simulink model "Pre_SysGen_Post_sh_fifo_nohwcs"  (Simulink 10.0)
settings: Solver=ode45  StartTime=0.0  StopTime=500000  RelTol=1e-3
InitFcn:
  | init
undefined symbols (not defined in the file): blk, cols, fps, rows
libraries: xbsIndex_r4 x178, simulink x14, dspbuff3 x6, dspmtrx3 x3, vipsnks x2, dspsrcs4 x2, dspsigops x1, dspwin32 x1
(part 1 of 2)
settings Model: Creator=ahwang  LastModifiedBy=bhisma
settings DataIOCC: LimitDataPoints=on  SignalLoggingSaveFormat=ModelDataLogs
settings OptimizationCC: ExpressionDepthLimit=2147483647  InitFltsAndDblsToZero=on
settings DebuggingCC: SaveWithParameterizedLinksMsg=none  SolverPrmCheckMsg=warning  FcnCallInpInsideContextMsg=warning  StateNameClashWarn=warning
settings SFSimCC: SimUseLocalCustomCode=on  CustomCodeUndefinedFunction=FilterOut
settings RTWCC: RTWUseLocalCustomCode=on
settings GRTTargetCC: TargetFcnLib=ansi_tfl_tmw.mat

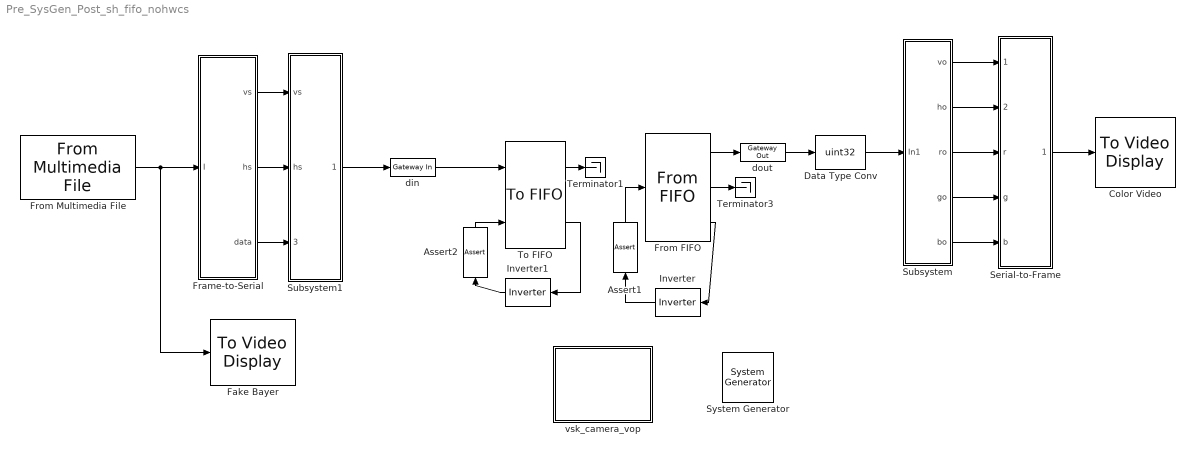
== system Pre_SysGen_Post_sh_fifo_nohwcs ==
  " System Generator" : xbsIndex_r4/ System Generator  Tag=genX  SystemSampleTime=-1  xilinxfamily=spartan3adsp  part=xc3sd1800a  speed=-4  package=fg676  synthesis_tool=XST  directory=./netlist  testbench=off  simulink_period=1  sysclk_period=20  incr_netlist=off  trim_vbits=Everywhere in SubSystem  dbl_ovrd=According to Block Masks  core_generation=According to Block Masks  run_coregen=off  deprecated_control=off  eval_field=0  block_type=sysgen
      settings: block_version=9.2.01
  Assert1 : xbsIndex_r4/Assert  assert_type=off  type_source=Explicitly  arith_type=Unsigned  n_bits=8  bin_pt=2  assert_rate=on  rate_source=Explicitly  period=1  output_port=on  block_type=assert
      settings: infoedit=Asserts a user-defined sample rate and/or type on a signal.  block_version=VER_STRING_GOES_HERE
  Assert2 : xbsIndex_r4/Assert  assert_type=off  type_source=Explicitly  arith_type=Unsigned  n_bits=8  bin_pt=2  assert_rate=on  rate_source=Explicitly  period=1  output_port=on  block_type=assert
      settings: infoedit=Asserts a user-defined sample rate and/or type on a signal.  block_version=VER_STRING_GOES_HERE
  Color Video : vipsnks/To Video Display  inputType=Obsolete  imagePorts=One multidimensional signal  OutputDevice=On-screen video monitor  fullScreen=off  videoWindowX=559  videoWindowY=678  saveWindowSize=off  videoWindowWidth=44  videoWindowHeight=41  dataOrg=Column-major
      settings: SourceProductName=Computer Vision Toolbox  SourceProductBaseCode=VP
  Data Type Conv : DataTypeConversion  OutDataTypeStr=uint32
  Fake Bayer : vipsnks/To Video Display  inputType=Obsolete  imagePorts=One multidimensional signal  OutputDevice=On-screen video monitor  fullScreen=off  videoWindowX=177  videoWindowY=679  saveWindowSize=off  videoWindowWidth=44  videoWindowHeight=41  dataOrg=Column-major
      settings: SourceProductName=Computer Vision Toolbox  SourceProductBaseCode=VP
  Frame-to-Serial : Subsystem
  From FIFO : xbsIndex_r4/From FIFO  shared_memory_name='data_out'  ownership=Owned elsewhere  depth=4K  percent_nbits=8  has_arst=off  arith_type=Unsigned  n_bits=32  bin_pt=0  dbl_ovrd=off  mem_type=Block RAM  block_type=fromfifo
      settings: AttributesFormatString=<< %<shared_memory_name> >>  infoedit=First-in-first-out (FIFO) block that reads FIFO data from shared memory storage.  block_version=VER_STRING_GOES_HERE
  From Multimedia File : dspwin32/From Multimedia File  inputFilename=C:\hill\WWM\seminars\mathworks_vsk\seminar_designs\viptrain_gbrg.avi  loop=on  numPlays=inf  outputStreams=Video only  videoDataType=uint8  audioDataType=int16  inheritSampleTime=off  userDefinedSampleTime=1/fps  noAudioOutput=off  isIntensityVideo=on  colorVideoFormat=One multidimensional signal  outputEOF=off  dataOrg=Column-major
      settings: SourceProductName=DSP System Toolbox  SourceProductBaseCode=DS
  Inverter : xbsIndex_r4/Inverter  en=off  latency=0  dbl_ovrd=off  block_type=inv
      settings: block_version=VER_STRING_GOES_HERE
  Inverter1 : xbsIndex_r4/Inverter  en=off  latency=0  dbl_ovrd=off  block_type=inv
      settings: block_version=VER_STRING_GOES_HERE
  Serial-to-Frame : Subsystem
  Subsystem : Subsystem
  Subsystem1 : Subsystem
  Terminator1 : Terminator
  Terminator3 : Terminator
  To FIFO : xbsIndex_r4/To FIFO  shared_memory_name='data_in'  ownership=Owned elsewhere  depth=16  percent_nbits=1  has_arst=off  explicit_data_type=on  arith_type=Unsigned  n_bits=16  bin_pt=0  dbl_ovrd=off  mem_type=Block RAM  block_type=tofifo
      settings: AttributesFormatString=<< %<shared_memory_name> >>  infoedit=First-in-first-out (FIFO) block that writes FIFO data to shared memory storage.  block_version=VER_STRING_GOES_HERE
  din : xbsIndex_r4/Gateway In  arith_type=Unsigned  n_bits=16  bin_pt=0  quantization="Round  (unbiased: +/- Inf)"  overflow=Saturate  period=1  dbl_ovrd=off  timing_constraint=None  locs_specified=off  LOCs={}  block_type=gatewayin
      settings: infoedit="Gateway in block.  Converts inputs of type Simulink integer, double and fixed point to  Xilinx fixed point type.<P><P>Hardware notes:  In hardware these blocks become top level input ports."  xl_area=[0, 0, 0, 0, 0, 0, 0]  block_version=VER_STRING_GOES_HERE
  dout : xbsIndex_r4/Gateway Out  hdl_port=on  timing_constraint=None  locs_specified=off  LOCs={}  block_type=gatewayout
      settings: infoedit="Gateway out block.  Converts Xilinx fixed point inputs into ouputs of type Simulink integer, double, or fixed point.<P><P>Hardware notes:  In hardware these blocks become top level output ports or are discarded, depending on how they are configured."  xl_area=[0, 0, 0, 0, 0, 0, 0]  block_version=VER_STRING_GOES_HERE
  vsk_camera_vop : Subsystem
  wires:
  From Multimedia File/1 -> Frame-to-Serial/1(I), Fake Bayer/1
  Serial-to-Frame/1(v_out) -> Color Video/1
  Frame-to-Serial/3(data) -> Subsystem1/3(data)
  Frame-to-Serial/2(hs) -> Subsystem1/2(hs)
  Frame-to-Serial/1(vs) -> Subsystem1/1(vs)
  Subsystem/5(bo) -> Serial-to-Frame/5(b)
  Subsystem/4(go) -> Serial-to-Frame/4(g)
  Subsystem/2(ho) -> Serial-to-Frame/2(hsync)
  Subsystem/1(vo) -> Serial-to-Frame/1(vsync)
  Subsystem/3(ro) -> Serial-to-Frame/3(r)
  From FIFO/1 -> dout/1
  din/1 -> To FIFO/1
  To FIFO/1 -> Terminator1/1
  To FIFO/2 -> Inverter1/1
  From FIFO/2 -> Terminator3/1
  From FIFO/3 -> Inverter/1
  Inverter/1 -> Assert1/1
  Assert2/1 -> To FIFO/2
  Assert1/1 -> From FIFO/1
  Inverter1/1 -> Assert2/1
  Subsystem1/1(Out1) -> din/1
  dout/1 -> Data Type Conv/1
  Data Type Conv/1 -> Subsystem/1(In1)

== system Pre_SysGen_Post_sh_fifo_nohwcs/Frame-to-Serial ==
  I : Inport
  Math Function : Math  Operator=transpose  SaturateOnIntegerOverflow=on
  Subsystem1 : Subsystem
  vs : Outport
  hs : Outport  Port=2
  data : Outport  Port=3
  wires:
  I/1 -> Math Function/1
  Math Function/1 -> Subsystem1/1(I)
  Subsystem1/1(vs) -> vs/1
  Subsystem1/2(hs) -> hs/1
  Subsystem1/3(data) -> data/1

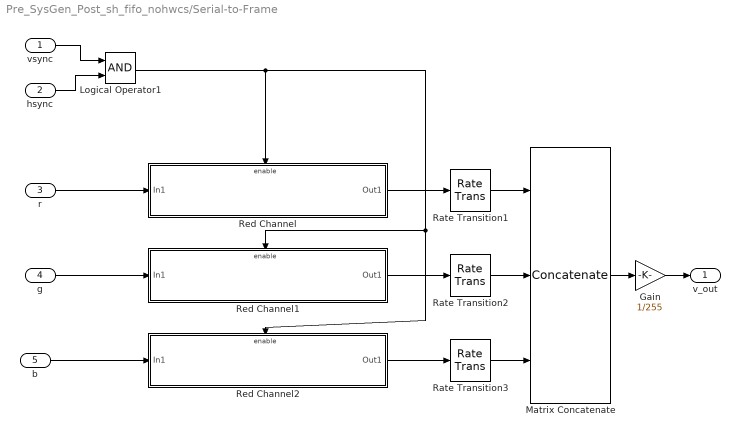
== system Pre_SysGen_Post_sh_fifo_nohwcs/Serial-to-Frame ==
  vsync : Inport
  hsync : Inport  Port=2
  r : Inport  Port=3
  g : Inport  Port=4
  b : Inport  Port=5
  Gain : Gain  Gain=1/255
  Logical Operator1 : Logic  AllPortsSameDT=off  OutDataTypeStr=boolean
  Matrix Concatenate : Concatenate  NumInputs=3  Mode=Multidimensional array  ConcatenateDimension=3
  Rate Transition1 : RateTransition  Deterministic=off  OutPortSampleTime=1/fps
  Rate Transition2 : RateTransition  Deterministic=off  OutPortSampleTime=1/fps
  Rate Transition3 : RateTransition  Deterministic=off  OutPortSampleTime=1/fps
  Red Channel : Subsystem
  Red Channel1 : Subsystem
  Red Channel2 : Subsystem
  v_out : Outport
  wires:
  Matrix Concatenate/1 -> Gain/1
  r/1 -> Red Channel/1(In1)
  g/1 -> Red Channel1/1(In1)
  b/1 -> Red Channel2/1(In1)
  Red Channel/1(Out1) -> Rate Transition1/1
  Red Channel1/1(Out1) -> Rate Transition2/1
  Red Channel2/1(Out1) -> Rate Transition3/1
  vsync/1 -> Logical Operator1/1
  hsync/1 -> Logical Operator1/2
  Logical Operator1/1 -> Red Channel/Enable, Red Channel1/Enable, Red Channel2/Enable
  Rate Transition1/1 -> Matrix Concatenate/1
  Rate Transition2/1 -> Matrix Concatenate/2
  Rate Transition3/1 -> Matrix Concatenate/3
  Gain/1 -> v_out/1

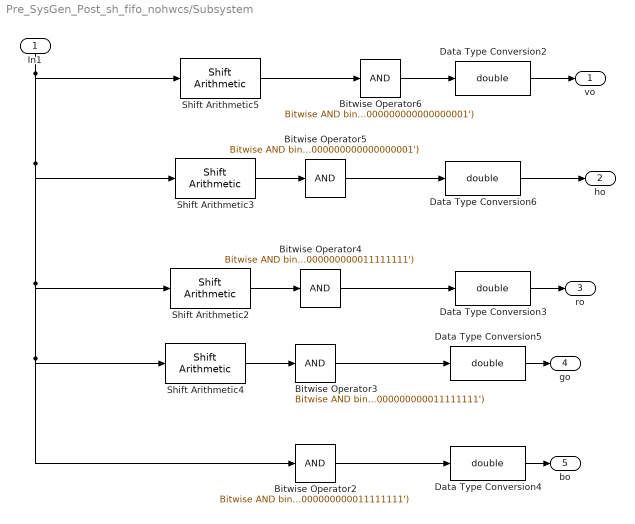
== system Pre_SysGen_Post_sh_fifo_nohwcs/Subsystem ==
  In1 : Inport
  Bitwise Operator2 : simulink/Logic and Bit Operations/Bitwise Operator  logicop=AND  UseBitMask=on  BitMask=bin2dec('000000000000000000011111111')  BitMaskRealWorld=Stored Integer
  Bitwise Operator3 : simulink/Logic and Bit Operations/Bitwise Operator  logicop=AND  UseBitMask=on  BitMask=bin2dec('000000000000000000011111111')  BitMaskRealWorld=Stored Integer
  Bitwise Operator4 : simulink/Logic and Bit Operations/Bitwise Operator  logicop=AND  UseBitMask=on  BitMask=bin2dec('000000000000000000011111111')  BitMaskRealWorld=Stored Integer
  Bitwise Operator5 : simulink/Logic and Bit Operations/Bitwise Operator  logicop=AND  UseBitMask=on  BitMask=bin2dec('000000000000000000000000001')  BitMaskRealWorld=Stored Integer
  Bitwise Operator6 : simulink/Logic and Bit Operations/Bitwise Operator  logicop=AND  UseBitMask=on  BitMask=bin2dec('000000000000000000000000001')  BitMaskRealWorld=Stored Integer
  Data Type Conversion{2..6} (5 alike) : DataTypeConversion  OutDataTypeStr=double
  Shift Arithmetic2 : simulink/Logic and Bit Operations/Shift Arithmetic  SystemSampleTime=-1  nBitShiftRight=16  nBinPtShiftRight=0
      settings: SourceProductName=Simulink  SourceProductBaseCode=SL
  Shift Arithmetic3 : simulink/Logic and Bit Operations/Shift Arithmetic  SystemSampleTime=-1  nBitShiftRight=24  nBinPtShiftRight=0
      settings: SourceProductName=Simulink  SourceProductBaseCode=SL
  Shift Arithmetic4 : simulink/Logic and Bit Operations/Shift Arithmetic  SystemSampleTime=-1  nBitShiftRight=8  nBinPtShiftRight=0
      settings: SourceProductName=Simulink  SourceProductBaseCode=SL
  Shift Arithmetic5 : simulink/Logic and Bit Operations/Shift Arithmetic  SystemSampleTime=-1  nBitShiftRight=25  nBinPtShiftRight=0
      settings: SourceProductName=Simulink  SourceProductBaseCode=SL
  vo : Outport
  ho : Outport  Port=2
  ro : Outport  Port=3
  go : Outport  Port=4
  bo : Outport  Port=5
  wires:
  Bitwise Operator5/1 -> Data Type Conversion6/1
  Bitwise Operator4/1 -> Data Type Conversion3/1
  Bitwise Operator3/1 -> Data Type Conversion5/1
  Shift Arithmetic5/1 -> Bitwise Operator6/1
  Shift Arithmetic3/1 -> Bitwise Operator5/1
  Shift Arithmetic2/1 -> Bitwise Operator4/1
  Shift Arithmetic4/1 -> Bitwise Operator3/1
  Bitwise Operator2/1 -> Data Type Conversion4/1
  In1/1 -> Shift Arithmetic5/1, Shift Arithmetic3/1, Shift Arithmetic2/1, Shift Arithmetic4/1, Bitwise Operator2/1
  Bitwise Operator6/1 -> Data Type Conversion2/1
  Data Type Conversion6/1 -> ho/1
  Data Type Conversion3/1 -> ro/1
  Data Type Conversion5/1 -> go/1
  Data Type Conversion4/1 -> bo/1
  Data Type Conversion2/1 -> vo/1

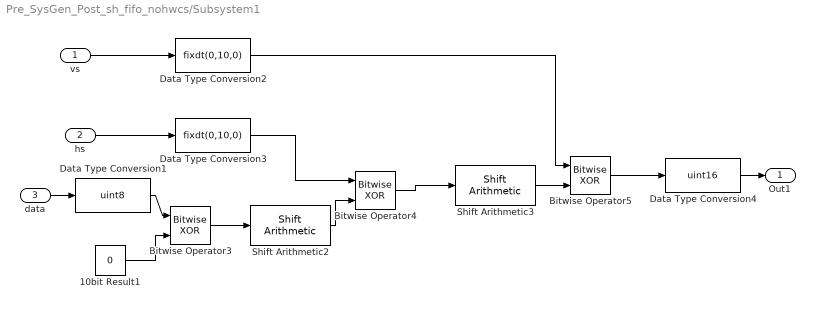
== system Pre_SysGen_Post_sh_fifo_nohwcs/Subsystem1 ==
  vs : Inport
  hs : Inport  Port=2
  data : Inport  Port=3
  10bit Result1 : Constant  Value=0  OutDataTypeStr=fixdt(0,10,0)
  Bitwise Operator3 : simulink/Logic and Bit Operations/Bitwise Operator  logicop=XOR  UseBitMask=off  NumInputPorts=2  BitMask=bin2dec('11011001')  BitMaskRealWorld=Stored Integer
  Bitwise Operator4 : simulink/Logic and Bit Operations/Bitwise Operator  logicop=XOR  UseBitMask=off  NumInputPorts=2  BitMask=bin2dec('11011001')  BitMaskRealWorld=Stored Integer
  Bitwise Operator5 : simulink/Logic and Bit Operations/Bitwise Operator  logicop=XOR  UseBitMask=off  NumInputPorts=2  BitMask=bin2dec('11011001')  BitMaskRealWorld=Stored Integer
  Data Type Conversion1 : DataTypeConversion  OutDataTypeStr=uint8
  Data Type Conversion2 : DataTypeConversion  OutDataTypeStr=fixdt(0,10,0)
  Data Type Conversion3 : DataTypeConversion  OutDataTypeStr=fixdt(0,10,0)
  Data Type Conversion4 : DataTypeConversion  OutDataTypeStr=uint16
  Shift Arithmetic2 : simulink/Logic and Bit Operations/Shift Arithmetic  SystemSampleTime=-1  nBitShiftRight=-1  nBinPtShiftRight=0
      settings: SourceProductName=Simulink  SourceProductBaseCode=SL
  Shift Arithmetic3 : simulink/Logic and Bit Operations/Shift Arithmetic  SystemSampleTime=-1  nBitShiftRight=-1  nBinPtShiftRight=0
      settings: SourceProductName=Simulink  SourceProductBaseCode=SL
  Out1 : Outport
  wires:
  10bit Result1/1 -> Bitwise Operator3/2
  Bitwise Operator3/1 -> Shift Arithmetic2/1
  Bitwise Operator4/1 -> Shift Arithmetic3/1
  Data Type Conversion1/1 -> Bitwise Operator3/1
  Shift Arithmetic2/1 -> Bitwise Operator4/2
  Data Type Conversion3/1 -> Bitwise Operator4/1
  Data Type Conversion2/1 -> Bitwise Operator5/1
  Shift Arithmetic3/1 -> Bitwise Operator5/2
  vs/1 -> Data Type Conversion2/1
  hs/1 -> Data Type Conversion3/1
  Bitwise Operator5/1 -> Data Type Conversion4/1
  data/1 -> Data Type Conversion1/1
  Data Type Conversion4/1 -> Out1/1

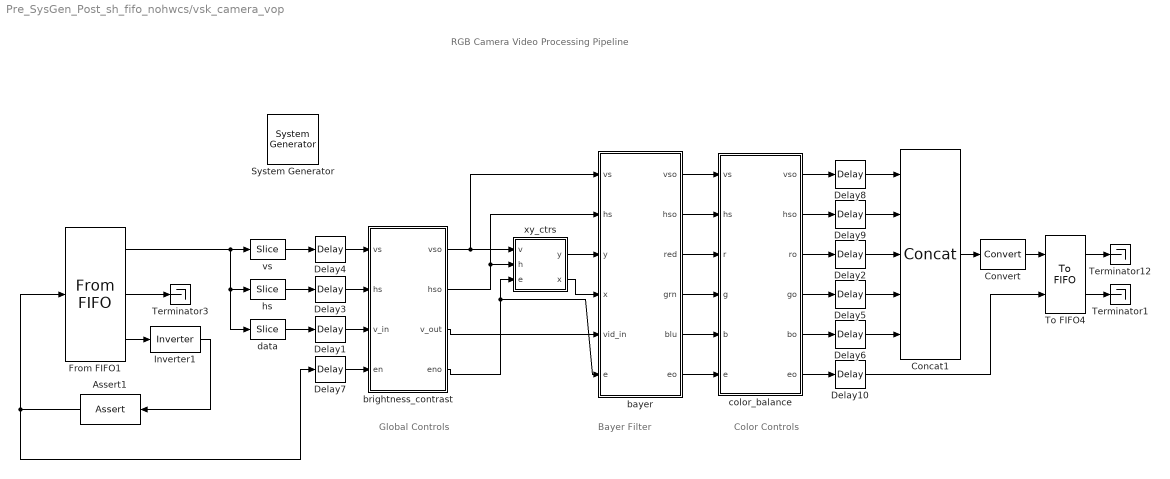
== system Pre_SysGen_Post_sh_fifo_nohwcs/vsk_camera_vop ==
  note: Color
      | Controls
  note: Global
      | Controls
  note: Bayer Filter
  note: RGB Camera Video Processing Pipeline
  " System Generator" : xbsIndex_r4/ System Generator  Tag=genX  SystemSampleTime=-1  xilinxfamily=spartan3adsp  part=xc3sd1800a  speed=-4  package=fg676  synthesis_tool=XST  directory=./netlist  testbench=off  simulink_period=1  sysclk_period=20  incr_netlist=off  trim_vbits=Everywhere in SubSystem  dbl_ovrd=According to Block Masks  core_generation=According to Block Masks  run_coregen=off  deprecated_control=off  eval_field=0  block_type=sysgen
      settings: block_version=9.2.01
  Assert1 : xbsIndex_r4/Assert  assert_type=off  type_source=Explicitly  arith_type=Unsigned  n_bits=8  bin_pt=2  assert_rate=on  rate_source=Explicitly  period=1  output_port=on  block_type=assert
      settings: infoedit=Asserts a user-defined sample rate and/or type on a signal.  block_version=VER_STRING_GOES_HERE
  Concat1 : xbsIndex_r4/Concat  num_inputs=5  dbl_ovrd=off  block_type=concat
      settings: block_version=9.2.01
  Convert : xbsIndex_r4/Convert  arith_type=Unsigned  n_bits=32  bin_pt=0  quantization=Truncate  overflow=Wrap  latency=0  dbl_ovrd=off  pipeline=off  block_type=convert
      settings: block_version=9.2.01
  Delay{1,3..4,7} (4 alike) : xbsIndex_r4/Delay  en=off  latency=20  dbl_ovrd=off  reg_retiming=on  block_type=delay
      settings: infoedit="Delay line having  configurable length.<P><P>Hardware notes: A delay line is a chain, each link of which is an SRL16 followed by a flip-flop. If register retiming is enabled, the delay line is a chain of flip-flops."  xl_area=[0, 0, 0, 0, 0, 0, 0]  block_version=VER_STRING_GOES_HERE
  Delay{2,5..6,8..10} (6 alike) : xbsIndex_r4/Delay  en=off  latency=1  dbl_ovrd=off  reg_retiming=on  block_type=delay
      settings: infoedit="Delay line having  configurable length.<P><P>Hardware notes: A delay line is a chain, each link of which is an SRL16 followed by a flip-flop. If register retiming is enabled, the delay line is a chain of flip-flops."  xl_area=[0, 0, 0, 0, 0, 0, 0]  block_version=VER_STRING_GOES_HERE
  From FIFO1 : xbsIndex_r4/From FIFO  shared_memory_name='data_in'  ownership=Locally owned  depth=64K  percent_nbits=1  has_arst=off  arith_type=Unsigned  n_bits=16  bin_pt=0  dbl_ovrd=off  mem_type=Block RAM  block_type=fromfifo
      settings: AttributesFormatString=<< %<shared_memory_name> >>  infoedit=First-in-first-out (FIFO) block that reads FIFO data from shared memory storage.  block_version=VER_STRING_GOES_HERE
  Inverter1 : xbsIndex_r4/Inverter  en=off  latency=0  dbl_ovrd=off  block_type=inv
      settings: block_version=VER_STRING_GOES_HERE
  Terminator1 : Terminator
  Terminator12 : Terminator
  Terminator3 : Terminator
  To FIFO4 : xbsIndex_r4/To FIFO  shared_memory_name='data_out'  ownership=Locally owned  depth=64K  percent_nbits=1  has_arst=off  explicit_data_type=on  arith_type=Unsigned  n_bits=32  bin_pt=0  dbl_ovrd=off  mem_type=Block RAM  block_type=tofifo
      settings: AttributesFormatString=<< %<shared_memory_name> >>  infoedit=First-in-first-out (FIFO) block that writes FIFO data to shared memory storage.  block_version=VER_STRING_GOES_HERE
  bayer : Subsystem
  brightness_contrast : Subsystem
  color_balance : Subsystem
  data : xbsIndex_r4/Slice  nbits=8  boolean_output=off  mode=Lower Bit Location + Width  bit1=0  base1=MSB of Input  bit0=2  base0=LSB of Input  dbl_ovrd=off  block_type=slice
      settings: infoedit="Extracts a given range of bits from each input sample and presents it at the output.  The output type is ordinarily unsigned with binary point at zero, but can be Boolean when the slice is one bit wide.<P><P>Hardware notes: In hardware this block costs nothing."  block_version=9.2.01
  hs : xbsIndex_r4/Slice  nbits=1  boolean_output=off  mode=Lower Bit Location + Width  bit1=0  base1=MSB of Input  bit0=1  base0=LSB of Input  dbl_ovrd=off  block_type=slice
      settings: infoedit="Extracts a given range of bits from each input sample and presents it at the output.  The output type is ordinarily unsigned with binary point at zero, but can be Boolean when the slice is one bit wide.<P><P>Hardware notes: In hardware this block costs nothing."  block_version=9.2.01
  vs : xbsIndex_r4/Slice  nbits=1  boolean_output=off  mode=Lower Bit Location + Width  bit1=0  base1=MSB of Input  bit0=0  base0=LSB of Input  dbl_ovrd=off  block_type=slice
      settings: infoedit="Extracts a given range of bits from each input sample and presents it at the output.  The output type is ordinarily unsigned with binary point at zero, but can be Boolean when the slice is one bit wide.<P><P>Hardware notes: In hardware this block costs nothing."  block_version=9.2.01
  xy_ctrs : Subsystem
  wires:
  Delay1/1 -> brightness_contrast/3(v_in)
  Delay3/1 -> brightness_contrast/2(hs)
  Delay4/1 -> brightness_contrast/1(vs)
  bayer/2(hso) -> color_balance/2(hs)
  bayer/1(vso) -> color_balance/1(vs)
  color_balance/2(hso) -> Delay9/1
  color_balance/1(vso) -> Delay8/1
  brightness_contrast/2(hso) -> bayer/2(hs), xy_ctrs/2(h)
  brightness_contrast/4(eno) -> xy_ctrs/3(e), bayer/6(e)
  brightness_contrast/1(vso) -> xy_ctrs/1(v), bayer/1(vs)
  Delay7/1 -> brightness_contrast/4(en)
  xy_ctrs/2(x) -> bayer/4(x)
  xy_ctrs/1(y) -> bayer/3(y)
  color_balance/5(bo) -> Delay6/1
  color_balance/4(go) -> Delay5/1
  color_balance/3(ro) -> Delay2/1
  bayer/6(eo) -> color_balance/6(e)
  bayer/5(blu) -> color_balance/5(b)
  bayer/4(grn) -> color_balance/4(g)
  bayer/3(red) -> color_balance/3(r)
  brightness_contrast/3(v_out) -> bayer/5(vid_in)
  From FIFO1/2 -> Terminator3/1
  From FIFO1/3 -> Inverter1/1
  From FIFO1/1 -> hs/1, data/1, vs/1
  To FIFO4/1 -> Terminator12/1
  vs/1 -> Delay4/1
  hs/1 -> Delay3/1
  data/1 -> Delay1/1
  To FIFO4/2 -> Terminator1/1
  Delay6/1 -> Concat1/5
  Delay5/1 -> Concat1/4
  Delay2/1 -> Concat1/3
  Delay9/1 -> Concat1/2
  Delay8/1 -> Concat1/1
  Concat1/1 -> Convert/1
  Inverter1/1 -> Assert1/1
  Assert1/1 -> From FIFO1/1, Delay7/1
  Convert/1 -> To FIFO4/1
  color_balance/6(eo) -> Delay10/1
  Delay10/1 -> To FIFO4/2

== system Pre_SysGen_Post_sh_fifo_nohwcs/Frame-to-Serial/Subsystem1 ==
  I : Inport
  Add : Sum
  Delay : dspsigops/Delay  dly_unit=Samples  delay=1  ic_detail=off  dif_ic_for_ch=off  dif_ic_for_dly=off  ic=0  reset_popup=Falling edge
      settings: SourceProductName=DSP System Toolbox  SourceProductBaseCode=DS
  Enabled Subsystem : Subsystem  TreatAsAtomicUnit=on
  Logical Operator : Logic  AllPortsSameDT=off  OutDataTypeStr=boolean
  Reshape : Reshape
  hsync : dspsrcs4/Signal From Workspace  SystemSampleTime=-1  X=[zeros(1,blk) ones(1,cols) zeros(1,blk)]  Ts=(1/fps)/ (rows*(cols+2*blk))  nsamps=1  OutputAfterFinalValue=Cyclic repetition  ignoreOrWarnInputAndFrameLengths=off
  vsync : dspsrcs4/Signal From Workspace  SystemSampleTime=-1  X=[ zeros(1,blk) ones(1,rows*(cols+2*blk)-2*blk) zeros(1,blk) ]  Ts=(1/fps)/(rows*(cols+2*blk))  nsamps=1  OutputAfterFinalValue=Cyclic repetition  ignoreOrWarnInputAndFrameLengths=off
  vs : Outport
  hs : Outport  Port=2
  data : Outport  Port=3
  wires:
  I/1 -> Reshape/1
  vsync/1 -> Delay/2, vs/1, Logical Operator/1  "Frame Valid"
  hsync/1 -> Add/2, hs/1, Logical Operator/2  "Line Valid"
  Delay/1 -> Add/1
  Add/1 -> Delay/1, Enabled Subsystem/2(Idx)
  Enabled Subsystem/1(Out1) -> data/1
  Reshape/1 -> Enabled Subsystem/1(I)
  Logical Operator/1 -> Enabled Subsystem/Enable

== system Pre_SysGen_Post_sh_fifo_nohwcs/Serial-to-Frame/Red Channel ==
  In1 : Inport
  Enable : EnablePort
  Buffer : dspbuff3/Buffer  N=cols  V=0  ic=0
      settings: SourceProductName=DSP System Toolbox  SourceProductBaseCode=DS
  Buffer1 : dspbuff3/Buffer  N=rows  V=0  ic=0
      settings: SourceProductName=DSP System Toolbox  SourceProductBaseCode=DS
  Frame Conversion1 : FrameConversion  OutFrame=Sample-based
  Matrix Concatenate : Concatenate  Mode=Multidimensional array
  Selector : Selector  NumberOfDimensions=2  InputPortWidth=3  IndexOptions=Index vector (dialog),Select all  Indices=22:rows,1  OutputSizes=1,1
  Selector1 : Selector  NumberOfDimensions=2  InputPortWidth=3  IndexOptions=Index vector (dialog),Select all  Indices=1:21,1  OutputSizes=1,1
  Transpose : dspmtrx3/Transpose  SystemSampleTime=-1  Hermitian=off  overflowFlag=off
      settings: SourceProductName=DSP System Toolbox  SourceProductBaseCode=DS
  Out1 : Outport
  wires:
  Buffer/1 -> Transpose/1
  In1/1 -> Buffer/1
  Transpose/1 -> Buffer1/1
  Frame Conversion1/1 -> Out1/1
  Matrix Concatenate/1 -> Frame Conversion1/1
  Selector/1 -> Matrix Concatenate/1
  Selector1/1 -> Matrix Concatenate/2
  Buffer1/1 -> Selector1/1, Selector/1

== system Pre_SysGen_Post_sh_fifo_nohwcs/Serial-to-Frame/Red Channel1 ==
  In1 : Inport
  Enable : EnablePort
  Buffer : dspbuff3/Buffer  N=cols  V=0  ic=0
      settings: SourceProductName=DSP System Toolbox  SourceProductBaseCode=DS
  Buffer1 : dspbuff3/Buffer  N=rows  V=0  ic=0
      settings: SourceProductName=DSP System Toolbox  SourceProductBaseCode=DS
  Frame Conversion1 : FrameConversion  OutFrame=Sample-based
  Matrix Concatenate : Concatenate  Mode=Multidimensional array
  Selector : Selector  NumberOfDimensions=2  InputPortWidth=3  IndexOptions=Index vector (dialog),Select all  Indices=22:rows,1  OutputSizes=1,1
  Selector1 : Selector  NumberOfDimensions=2  InputPortWidth=3  IndexOptions=Index vector (dialog),Select all  Indices=1:21,1  OutputSizes=1,1
  Transpose : dspmtrx3/Transpose  SystemSampleTime=-1  Hermitian=off  overflowFlag=off
      settings: SourceProductName=DSP System Toolbox  SourceProductBaseCode=DS
  Out1 : Outport
  wires:
  Buffer1/1 -> Selector/1, Selector1/1
  Selector1/1 -> Matrix Concatenate/2
  Selector/1 -> Matrix Concatenate/1
  Matrix Concatenate/1 -> Frame Conversion1/1
  Frame Conversion1/1 -> Out1/1
  Transpose/1 -> Buffer1/1
  In1/1 -> Buffer/1
  Buffer/1 -> Transpose/1

== system Pre_SysGen_Post_sh_fifo_nohwcs/Serial-to-Frame/Red Channel2 ==
  In1 : Inport
  Enable : EnablePort
  Buffer : dspbuff3/Buffer  N=cols  V=0  ic=0
      settings: SourceProductName=DSP System Toolbox  SourceProductBaseCode=DS
  Buffer1 : dspbuff3/Buffer  N=rows  V=0  ic=0
      settings: SourceProductName=DSP System Toolbox  SourceProductBaseCode=DS
  Frame Conversion1 : FrameConversion  OutFrame=Sample-based
  Matrix Concatenate : Concatenate  Mode=Multidimensional array
  Selector : Selector  NumberOfDimensions=2  InputPortWidth=3  IndexOptions=Index vector (dialog),Select all  Indices=22:rows,1  OutputSizes=1,1
  Selector1 : Selector  NumberOfDimensions=2  InputPortWidth=3  IndexOptions=Index vector (dialog),Select all  Indices=1:21,1  OutputSizes=1,1
  Transpose : dspmtrx3/Transpose  SystemSampleTime=-1  Hermitian=off  overflowFlag=off
      settings: SourceProductName=DSP System Toolbox  SourceProductBaseCode=DS
  Out1 : Outport
  wires:
  Buffer/1 -> Transpose/1
  In1/1 -> Buffer/1
  Transpose/1 -> Buffer1/1
  Frame Conversion1/1 -> Out1/1
  Matrix Concatenate/1 -> Frame Conversion1/1
  Selector/1 -> Matrix Concatenate/1
  Selector1/1 -> Matrix Concatenate/2
  Buffer1/1 -> Selector1/1, Selector/1

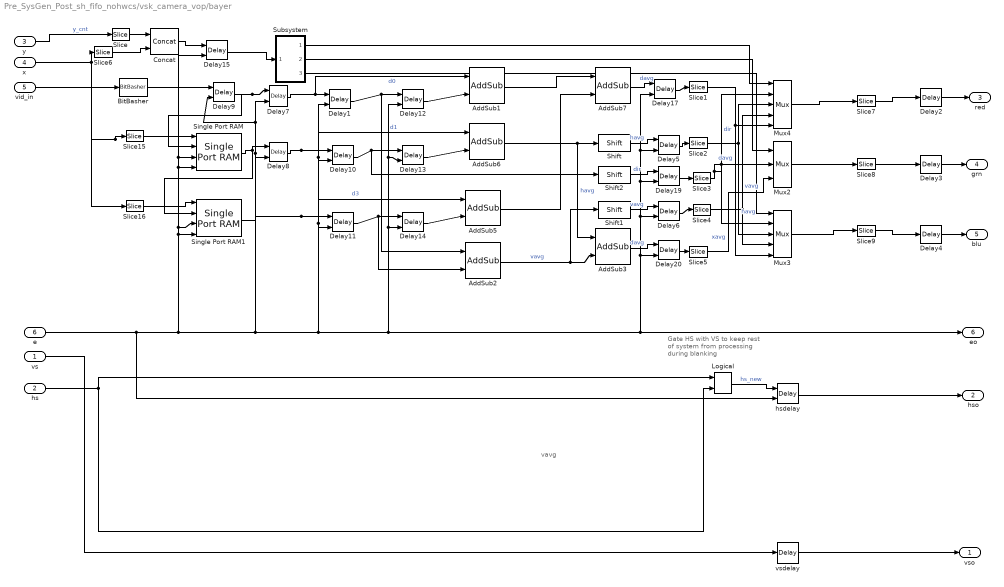
== system Pre_SysGen_Post_sh_fifo_nohwcs/vsk_camera_vop/bayer ==
  note: Gate HS with VS to keep
      | rest of system from
      | processing during blanking
  note: vavg
  vs : Inport
  hs : Inport  Port=2
  y : Inport  Port=3
  x : Inport  Port=4
  vid_in : Inport  Port=5
  e : Inport  Port=6
  AddSub{1..3,5..7} (6 alike) : xbsIndex_r4/AddSub  mode=Addition  use_carryin=off  use_carryout=off  en=off  latency=0  precision=Full  arith_type=Unsigned  n_bits=8  bin_pt=2  quantization=Truncate  overflow=Wrap  dbl_ovrd=off  use_behavioral_HDL=off  pipelined=off  use_rpm=on  block_type=addsub
      settings: xl_area=[0, 0, 0, 0, 0, 0, 0]  block_version=VER_STRING_GOES_HERE
  BitBasher : xbsIndex_r4/BitBasher  bitexpr=|  display_expr=off  sr_1=1  arith_type1=Unsigned  bin_pt1=0  sr_2=2  arith_type2=Unsigned  bin_pt2=0  sr_3=3  arith_type3=Unsigned  bin_pt3=0  sr_4=4  arith_type4=Unsigned  bin_pt4=0  dbl_ovrd=off  block_type=bitbasher
      | <html><head><meta name="qrichtext" content="1" /><style type="text/css">
      | p, li { white-space: pre-wrap; }
      | </style></head><body style=" font-family:'MS Shell Dlg 2'; font-size:8.25pt; font-weight:400; font-style:normal;">
      | <p style=" margin-top:12px; margin-bottom:12px; margin-left:0px; margin-right:0px; -qt-block-indent:0; text-indent:0px; font-family:'MS Shell Dlg'; font-size:8pt;">pad={in,2'b00}</p></body></html>
      settings: block_version=9.2.01
  Concat : xbsIndex_r4/Concat  num_inputs=2  dbl_ovrd=off  block_type=concat
      settings: block_version=VER_STRING_GOES_HERE
  Delay{1,5..6,8,10..15,17,19..20} (13 alike) : xbsIndex_r4/Delay  en=on  latency=1  dbl_ovrd=off  reg_retiming=on  block_type=delay
      settings: infoedit="Delay line having  configurable length.<P><P>Hardware notes: A delay line is a chain, each link of which is an SRL16 followed by a flip-flop. If register retiming is enabled, the delay line is a chain of flip-flops."  xl_area=[0, 0, 0, 0, 0, 0, 0]  block_version=VER_STRING_GOES_HERE
  Delay2 : xbsIndex_r4/Delay  en=off  latency=1  dbl_ovrd=off  reg_retiming=on  block_type=delay
      settings: infoedit="Delay line having  configurable length.<P><P>Hardware notes: A delay line is a chain, each link of which is an SRL16 followed by a flip-flop. If register retiming is enabled, the delay line is a chain of flip-flops."  xl_area=[0, 0, 0, 0, 0, 0, 0]  block_version=VER_STRING_GOES_HERE
  Delay3 : xbsIndex_r4/Delay  en=off  latency=1  dbl_ovrd=off  reg_retiming=on  block_type=delay
      settings: infoedit="Delay line having  configurable length.<P><P>Hardware notes: A delay line is a chain, each link of which is an SRL16 followed by a flip-flop. If register retiming is enabled, the delay line is a chain of flip-flops."  xl_area=[0, 0, 0, 0, 0, 0, 0]  block_version=VER_STRING_GOES_HERE
  Delay4 : xbsIndex_r4/Delay  en=off  latency=1  dbl_ovrd=off  reg_retiming=on  block_type=delay
      settings: infoedit="Delay line having  configurable length.<P><P>Hardware notes: A delay line is a chain, each link of which is an SRL16 followed by a flip-flop. If register retiming is enabled, the delay line is a chain of flip-flops."  xl_area=[0, 0, 0, 0, 0, 0, 0]  block_version=VER_STRING_GOES_HERE
  Delay7 : xbsIndex_r4/Delay  en=on  latency=2  dbl_ovrd=off  reg_retiming=on  block_type=delay
      settings: infoedit="Delay line having  configurable length.<P><P>Hardware notes: A delay line is a chain, each link of which is an SRL16 followed by a flip-flop. If register retiming is enabled, the delay line is a chain of flip-flops."  xl_area=[0, 0, 0, 0, 0, 0, 0]  block_version=VER_STRING_GOES_HERE
  Delay9 : xbsIndex_r4/Delay  en=on  latency=2  dbl_ovrd=off  reg_retiming=on  block_type=delay
      settings: infoedit="Delay line having  configurable length.<P><P>Hardware notes: A delay line is a chain, each link of which is an SRL16 followed by a flip-flop. If register retiming is enabled, the delay line is a chain of flip-flops."  xl_area=[0, 0, 0, 0, 0, 0, 0]  block_version=VER_STRING_GOES_HERE
  Logical : xbsIndex_r4/Logical  logical_function=AND  inputs=2  en=off  latency=0  precision=Full  arith_type=Unsigned  n_bits=16  bin_pt=0  align_bp=on  dbl_ovrd=off  block_type=logical
      settings: block_version=9.2.01
  Mux2 : xbsIndex_r4/Mux  inputs=2  en=off  latency=0  precision=Full  arith_type="Signed  (2's comp)"  n_bits=8  bin_pt=2  quantization=Truncate  overflow=Wrap  dbl_ovrd=off  block_type=mux
      settings: xl_area=[0, 0, 0, 0, 0, 0, 0]  block_version=VER_STRING_GOES_HERE
  Mux3 : xbsIndex_r4/Mux  inputs=4  en=off  latency=0  precision=Full  arith_type="Signed  (2's comp)"  n_bits=8  bin_pt=2  quantization=Truncate  overflow=Wrap  dbl_ovrd=off  block_type=mux
      settings: xl_area=[0, 0, 0, 0, 0, 0, 0]  block_version=VER_STRING_GOES_HERE
  Mux4 : xbsIndex_r4/Mux  inputs=4  en=off  latency=0  precision=Full  arith_type="Signed  (2's comp)"  n_bits=8  bin_pt=2  quantization=Truncate  overflow=Wrap  dbl_ovrd=off  block_type=mux
      settings: xl_area=[0, 0, 0, 0, 0, 0, 0]  block_version=VER_STRING_GOES_HERE
  Shift : xbsIndex_r4/Shift  shift_dir=Left  shift_bits=1  en=off  latency=0  precision=User Defined  arith_type=Unsigned  n_bits=12  bin_pt=0  quantization=Truncate  overflow=Wrap  dbl_ovrd=off  block_type=shift
      settings: xl_area=[0, 0, 0, 0, 0, 0, 0]  block_version=VER_STRING_GOES_HERE
  Shift1 : xbsIndex_r4/Shift  shift_dir=Left  shift_bits=1  en=off  latency=0  precision=User Defined  arith_type=Unsigned  n_bits=12  bin_pt=0  quantization=Truncate  overflow=Wrap  dbl_ovrd=off  block_type=shift
      settings: xl_area=[0, 0, 0, 0, 0, 0, 0]  block_version=VER_STRING_GOES_HERE
  Shift2 : xbsIndex_r4/Shift  shift_dir=Left  shift_bits=2  en=off  latency=0  precision=User Defined  arith_type=Unsigned  n_bits=12  bin_pt=0  quantization=Truncate  overflow=Wrap  dbl_ovrd=off  block_type=shift
      settings: xl_area=[0, 0, 0, 0, 0, 0, 0]  block_version=VER_STRING_GOES_HERE
  Single Port RAM : xbsIndex_r4/Single Port RAM  depth=1024  initVector=0  distributed_mem=Block RAM  write_mode=Read Before Write  rst=off  init_reg=0  en=on  latency=1  dbl_ovrd=off  optimize=Area  use_rpm=off  block_type=spram
      settings: xl_area=[0, 0, 0, 0, 0, 0, 0]  block_version=8.2
  Single Port RAM1 : xbsIndex_r4/Single Port RAM  depth=1024  initVector=0  distributed_mem=Block RAM  write_mode=Read Before Write  rst=off  init_reg=0  en=on  latency=1  dbl_ovrd=off  optimize=Area  use_rpm=off  block_type=spram
      settings: xl_area=[0, 0, 0, 0, 0, 0, 0]  block_version=8.2
  Slice : xbsIndex_r4/Slice  nbits=1  boolean_output=off  mode=Lower Bit Location + Width  bit1=0  base1=MSB of Input  bit0=0  base0=LSB of Input  dbl_ovrd=off  block_type=slice
      settings: infoedit="Extracts a given range of bits from each input sample and presents it at the output.  The output type is ordinarily unsigned with binary point at zero, but can be Boolean when the slice is one bit wide.<P><P>Hardware notes: In hardware this block costs nothing."  block_version=VER_STRING_GOES_HERE
  Slice{1..5} (5 alike) : xbsIndex_r4/Slice  nbits=10  boolean_output=off  mode=Lower Bit Location + Width  bit1=0  base1=MSB of Input  bit0=2  base0=LSB of Input  dbl_ovrd=off  block_type=slice
      settings: infoedit="Extracts a given range of bits from each input sample and presents it at the output.  The output type is ordinarily unsigned with binary point at zero, but can be Boolean when the slice is one bit wide.<P><P>Hardware notes: In hardware this block costs nothing."  block_version=VER_STRING_GOES_HERE
  Slice15 : xbsIndex_r4/Slice  nbits=10  boolean_output=off  mode=Lower Bit Location + Width  bit1=0  base1=MSB of Input  bit0=0  base0=LSB of Input  dbl_ovrd=off  block_type=slice
      settings: infoedit="Extracts a given range of bits from each input sample and presents it at the output.  The output type is ordinarily unsigned with binary point at zero, but can be Boolean when the slice is one bit wide.<P><P>Hardware notes: In hardware this block costs nothing."  block_version=VER_STRING_GOES_HERE
  Slice16 : xbsIndex_r4/Slice  nbits=10  boolean_output=off  mode=Lower Bit Location + Width  bit1=0  base1=MSB of Input  bit0=0  base0=LSB of Input  dbl_ovrd=off  block_type=slice
      settings: infoedit="Extracts a given range of bits from each input sample and presents it at the output.  The output type is ordinarily unsigned with binary point at zero, but can be Boolean when the slice is one bit wide.<P><P>Hardware notes: In hardware this block costs nothing."  block_version=VER_STRING_GOES_HERE
  Slice6 : xbsIndex_r4/Slice  nbits=1  boolean_output=off  mode=Lower Bit Location + Width  bit1=0  base1=MSB of Input  bit0=0  base0=LSB of Input  dbl_ovrd=off  block_type=slice
      settings: infoedit="Extracts a given range of bits from each input sample and presents it at the output.  The output type is ordinarily unsigned with binary point at zero, but can be Boolean when the slice is one bit wide.<P><P>Hardware notes: In hardware this block costs nothing."  block_version=VER_STRING_GOES_HERE
  Slice7 : xbsIndex_r4/Slice  nbits=8  boolean_output=off  mode=Lower Bit Location + Width  bit1=0  base1=MSB of Input  bit0=2  base0=LSB of Input  dbl_ovrd=off  block_type=slice
      settings: infoedit="Extracts a given range of bits from each input sample and presents it at the output.  The output type is ordinarily unsigned with binary point at zero, but can be Boolean when the slice is one bit wide.<P><P>Hardware notes: In hardware this block costs nothing."  block_version=VER_STRING_GOES_HERE
  Slice8 : xbsIndex_r4/Slice  nbits=8  boolean_output=off  mode=Lower Bit Location + Width  bit1=0  base1=MSB of Input  bit0=2  base0=LSB of Input  dbl_ovrd=off  block_type=slice
      settings: infoedit="Extracts a given range of bits from each input sample and presents it at the output.  The output type is ordinarily unsigned with binary point at zero, but can be Boolean when the slice is one bit wide.<P><P>Hardware notes: In hardware this block costs nothing."  block_version=VER_STRING_GOES_HERE
  Slice9 : xbsIndex_r4/Slice  nbits=8  boolean_output=off  mode=Lower Bit Location + Width  bit1=0  base1=MSB of Input  bit0=2  base0=LSB of Input  dbl_ovrd=off  block_type=slice
      settings: infoedit="Extracts a given range of bits from each input sample and presents it at the output.  The output type is ordinarily unsigned with binary point at zero, but can be Boolean when the slice is one bit wide.<P><P>Hardware notes: In hardware this block costs nothing."  block_version=VER_STRING_GOES_HERE
  Subsystem : Subsystem
  hsdelay : xbsIndex_r4/Delay  en=on  latency=7  dbl_ovrd=off  reg_retiming=on  block_type=delay
      settings: infoedit="Delay line having  configurable length.<P><P>Hardware notes: A delay line is a chain, each link of which is an SRL16 followed by a flip-flop. If register retiming is enabled, the delay line is a chain of flip-flops."  xl_area=[0, 0, 0, 0, 0, 0, 0]  block_version=VER_STRING_GOES_HERE
  vsdelay : xbsIndex_r4/Delay  en=off  latency=7  dbl_ovrd=off  reg_retiming=on  block_type=delay
      settings: infoedit="Delay line having  configurable length.<P><P>Hardware notes: A delay line is a chain, each link of which is an SRL16 followed by a flip-flop. If register retiming is enabled, the delay line is a chain of flip-flops."  xl_area=[0, 0, 0, 0, 0, 0, 0]  block_version=VER_STRING_GOES_HERE
  vso : Outport
  hso : Outport  Port=2
  red : Outport  Port=3
  grn : Outport  Port=4
  blu : Outport  Port=5
  eo : Outport  Port=6
  wires:
  Logical/1 -> hsdelay/1  "hs_new"
  vs/1 -> vsdelay/1
  e/1 -> hsdelay/2, Single Port RAM1/4, Delay15/2, Single Port RAM/3, Single Port RAM/4, Single Port RAM1/3, Delay10/2, Delay1/2, Delay11/2, Delay20/2, Delay6/2, Delay19/2, Delay5/2, Delay17/2, eo/1, Delay13/2, Delay12/2, Delay14/2, Delay7/2, Delay9/2, Delay8/2
  hs/1 -> Logical/1, Logical/2
  Slice9/1 -> Delay4/1
  Slice8/1 -> Delay3/1
  Slice7/1 -> Delay2/1
  vid_in/1 -> BitBasher/1
  BitBasher/1 -> Delay9/1
  Slice4/1 -> Mux3/4, Mux4/4  "vavg"
  Slice2/1 -> Mux3/3, Mux4/3  "havg"
  Slice1/1 -> Mux3/5, Mux4/5  "davg"
  Concat/1 -> Delay15/1
  Delay15/1 -> Subsystem/1(pos)
  Slice6/1 -> Concat/2
  Slice/1 -> Concat/1
  Slice5/1 -> Mux2/3  "xavg"
  Slice3/1 -> Mux3/2, Mux2/2, Mux4/2  "dir"
  Delay8/1 -> AddSub6/1, Delay10/1  "d1"
  Delay7/1 -> AddSub1/1, Delay1/1  "d0"
  x/1 -> Slice6/1, Slice15/1, Slice16/1
  Shift2/1 -> Delay19/1  "dir"
  Shift1/1 -> Delay6/1  "vavg"
  Shift/1 -> Delay5/1  "havg"
  Delay20/1 -> Slice5/1
  AddSub3/1 -> Delay20/1  "davg"
  Delay5/1 -> Slice2/1
  Delay19/1 -> Slice3/1
  Delay6/1 -> Slice4/1
  AddSub2/1 -> Shift1/1, AddSub3/2  "vavg"
  Subsystem/2(gsel) -> Mux2/1
  Slice16/1 -> Single Port RAM1/1
  Slice15/1 -> Single Port RAM/1
  Subsystem/1(rsel) -> Mux4/1
  Delay4/1 -> blu/1
  Delay3/1 -> grn/1
  Delay2/1 -> red/1
  Mux3/1 -> Slice9/1
  Mux2/1 -> Slice8/1
  Mux4/1 -> Slice7/1
  Subsystem/3(bsel) -> Mux3/1
  y/1 -> Slice/1  "y_cnt"
  AddSub6/1 -> Shift/1, AddSub3/1  "havg"
  Delay17/1 -> Slice1/1
  AddSub7/1 -> Delay17/1  "davg"
  AddSub5/1 -> AddSub7/2
  AddSub1/1 -> AddSub7/1
  Delay13/1 -> AddSub6/2
  Delay14/1 -> AddSub5/2
  Delay12/1 -> AddSub1/2
  Delay11/1 -> AddSub2/2, Delay14/1
  Delay10/1 -> Shift2/1, Delay13/1
  Delay1/1 -> AddSub2/1, Delay12/1
  Single Port RAM1/1 -> AddSub5/1, Delay11/1  "d3"
  Delay9/1 -> Delay7/1, Single Port RAM/2
  Single Port RAM/1 -> Single Port RAM1/2, Delay8/1
  hsdelay/1 -> hso/1
  vsdelay/1 -> vso/1

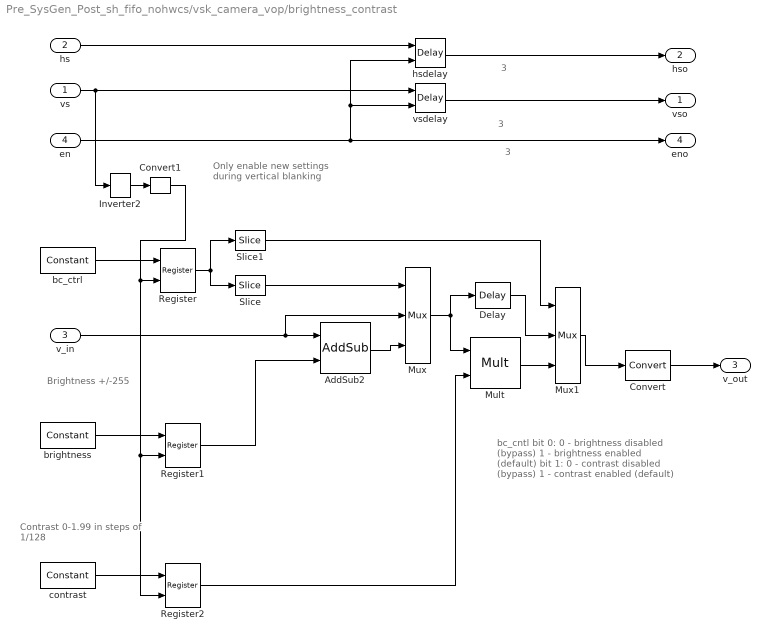
== system Pre_SysGen_Post_sh_fifo_nohwcs/vsk_camera_vop/brightness_contrast ==
  note: Only enable new settings
      | during vertical blanking
  note: bc_cntl
      | bit 0: 0 - brightness disabled (bypass)
      | 1 - brightness enabled (default)
      | bit 1: 0 - contrast disabled (bypass)
      | 1 - contrast enabled (default)
  note: Contrast
      | 0-1.99 in steps of 1/128
  note: Brightness
      | +/-255
  note: 3
  note: 3
  note: 3
  vs : Inport
  hs : Inport  Port=2
  v_in : Inport  Port=3
  en : Inport  Port=4
  AddSub2 : xbsIndex_r4/AddSub  mode=Addition  use_carryin=off  use_carryout=off  en=off  latency=0  precision=Full  arith_type=Unsigned  n_bits=8  bin_pt=2  quantization=Truncate  overflow=Wrap  dbl_ovrd=off  use_behavioral_HDL=off  pipelined=off  use_rpm=on  block_type=addsub
      settings: xl_area=[0, 0, 0, 0, 0, 0, 0]  block_version=VER_STRING_GOES_HERE
  Convert : xbsIndex_r4/Convert  arith_type=Unsigned  n_bits=8  bin_pt=0  quantization="Round  (unbiased: +/- Inf)"  overflow=Saturate  latency=0  dbl_ovrd=off  pipeline=off  block_type=convert
      settings: block_version=9.2.01
  Convert1 : xbsIndex_r4/Convert  arith_type=Boolean  n_bits=16  bin_pt=14  quantization=Truncate  overflow=Wrap  latency=0  dbl_ovrd=off  pipeline=off  block_type=convert
      settings: block_version=9.2.01
  Delay : xbsIndex_r4/Delay  en=off  latency=3  dbl_ovrd=off  reg_retiming=off  block_type=delay
      settings: block_version=9.2.01
  Inverter2 : xbsIndex_r4/Inverter  en=off  latency=0  dbl_ovrd=off  block_type=inv
      settings: block_version=9.2.01
  Mult : xbsIndex_r4/Mult  precision=Full  arith_type="Signed  (2's comp)"  n_bits=8  bin_pt=2  quantization=Truncate  overflow=Wrap  en=off  latency=3  dbl_ovrd=off  use_behavioral_HDL=off  use_embedded=on  opt=Speed  optimum_pipeline=off  pipeline=on  use_rpm=on  placement_style=Rectangular shape  block_type=mult
      settings: infoedit=Multiplies two values.<P><P>Hardware notes: To use the internal pipeline stage of the dedicated multiplier you must select 'Pipeline to Greatest Extent Possible'.  xl_area=[0, 0, 0, 0, 0, 0, 0]  block_version=VER_STRING_GOES_HERE
  Mux : xbsIndex_r4/Mux  inputs=2  en=off  latency=0  precision=Full  arith_type=Unsigned  n_bits=16  bin_pt=14  quantization=Truncate  overflow=Wrap  dbl_ovrd=off  block_type=mux
      settings: block_version=9.2.01
  Mux1 : xbsIndex_r4/Mux  inputs=2  en=off  latency=0  precision=Full  arith_type=Unsigned  n_bits=16  bin_pt=14  quantization=Truncate  overflow=Wrap  dbl_ovrd=off  block_type=mux
      settings: block_version=9.2.01
  Register : xbsIndex_r4/Register  init=0  rst=off  en=on  dbl_ovrd=off  block_type=register
      settings: block_version=9.2.01
  Register1 : xbsIndex_r4/Register  init=0  rst=off  en=on  dbl_ovrd=off  block_type=register
      settings: block_version=9.2.01
  Register2 : xbsIndex_r4/Register  init=0  rst=off  en=on  dbl_ovrd=off  block_type=register
      settings: block_version=9.2.01
  Slice : xbsIndex_r4/Slice  nbits=1  boolean_output=off  mode=Lower Bit Location + Width  bit1=0  base1=MSB of Input  bit0=0  base0=LSB of Input  dbl_ovrd=off  block_type=slice
      settings: infoedit="Extracts a given range of bits from each input sample and presents it at the output.  The output type is ordinarily unsigned with binary point at zero, but can be Boolean when the slice is one bit wide.<P><P>Hardware notes: In hardware this block costs nothing."  block_version=9.2.01
  Slice1 : xbsIndex_r4/Slice  nbits=1  boolean_output=off  mode=Lower Bit Location + Width  bit1=0  base1=MSB of Input  bit0=1  base0=LSB of Input  dbl_ovrd=off  block_type=slice
      settings: infoedit="Extracts a given range of bits from each input sample and presents it at the output.  The output type is ordinarily unsigned with binary point at zero, but can be Boolean when the slice is one bit wide.<P><P>Hardware notes: In hardware this block costs nothing."  block_version=9.2.01
  bc_ctrl : xbsIndex_r4/Constant  arith_type=Unsigned  const=0  n_bits=9  bin_pt=0  explicit_period=off  period=1  equ=P=C  opselect=C  inp2=PCIN>>17  opr=+  inp1=P  carry=CIN  dbl_ovrd=off  block_type=constant
      settings: block_version=9.2.01
  brightness : xbsIndex_r4/Constant  arith_type=Signed (2's comp)  const=0  n_bits=9  bin_pt=0  explicit_period=off  period=1  equ=P=C  opselect=C  inp2=PCIN>>17  opr=+  inp1=P  carry=CIN  dbl_ovrd=off  block_type=constant
      settings: block_version=9.2.01
  contrast : xbsIndex_r4/Constant  arith_type=Unsigned  const=8  n_bits=7  bin_pt=0  explicit_period=off  period=1  equ=P=C  opselect=C  inp2=PCIN>>17  opr=+  inp1=P  carry=CIN  dbl_ovrd=off  block_type=constant
      settings: block_version=9.2.01
  hsdelay : xbsIndex_r4/Delay  en=on  latency=3  dbl_ovrd=off  reg_retiming=on  block_type=delay
      settings: infoedit="Delay line having  configurable length.<P><P>Hardware notes: A delay line is a chain, each link of which is an SRL16 followed by a flip-flop. If register retiming is enabled, the delay line is a chain of flip-flops."  xl_area=[0, 0, 0, 0, 0, 0, 0]  block_version=VER_STRING_GOES_HERE
  vsdelay : xbsIndex_r4/Delay  en=on  latency=3  dbl_ovrd=off  reg_retiming=on  block_type=delay
      settings: infoedit="Delay line having  configurable length.<P><P>Hardware notes: A delay line is a chain, each link of which is an SRL16 followed by a flip-flop. If register retiming is enabled, the delay line is a chain of flip-flops."  xl_area=[0, 0, 0, 0, 0, 0, 0]  block_version=VER_STRING_GOES_HERE
  vso : Outport
  hso : Outport  Port=2
  v_out : Outport  Port=3
  eno : Outport  Port=4
  wires:
  hs/1 -> hsdelay/1
  Convert1/1 -> Register1/2, Register2/2, Register/2
  Inverter2/1 -> Convert1/1
  Register2/1 -> Mult/2
  Register1/1 -> AddSub2/2
  contrast/1 -> Register2/1
  brightness/1 -> Register1/1
  Register/1 -> Slice1/1, Slice/1
  bc_ctrl/1 -> Register/1
  Delay/1 -> Mux1/2
  Slice1/1 -> Mux1/1
  Mux1/1 -> Convert/1
  Mult/1 -> Mux1/3
  Slice/1 -> Mux/1
  Mux/1 -> Delay/1, Mult/1
  AddSub2/1 -> Mux/3
  en/1 -> vsdelay/2, hsdelay/2, eno/1
  vs/1 -> Inverter2/1, vsdelay/1
  v_in/1 -> Mux/2, AddSub2/1
  Convert/1 -> v_out/1
  hsdelay/1 -> hso/1
  vsdelay/1 -> vso/1

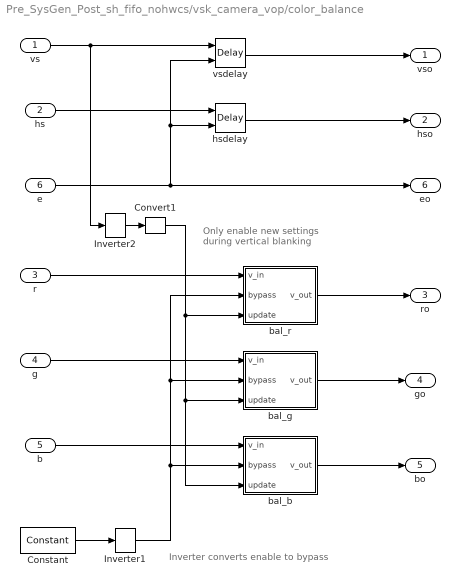
== system Pre_SysGen_Post_sh_fifo_nohwcs/vsk_camera_vop/color_balance ==
  note: Inverter converts enable to bypass
  note: Only enable new settings
      | during vertical blanking
  vs : Inport
  hs : Inport  Port=2
  r : Inport  Port=3
  g : Inport  Port=4
  b : Inport  Port=5
  e : Inport  Port=6
  Constant : xbsIndex_r4/Constant  arith_type=Unsigned  const=1  n_bits=1  bin_pt=0  explicit_period=off  period=1  equ=P=C  opselect=C  inp2=PCIN>>17  opr=+  inp1=P  carry=CIN  dbl_ovrd=off  block_type=constant
      settings: block_version=9.2.01
  Convert1 : xbsIndex_r4/Convert  arith_type=Boolean  n_bits=16  bin_pt=14  quantization=Truncate  overflow=Wrap  latency=0  dbl_ovrd=off  pipeline=off  block_type=convert
      settings: block_version=9.2.01
  Inverter1 : xbsIndex_r4/Inverter  en=off  latency=0  dbl_ovrd=off  block_type=inv
      settings: block_version=9.2.01
  Inverter2 : xbsIndex_r4/Inverter  en=off  latency=0  dbl_ovrd=off  block_type=inv
      settings: block_version=9.2.01
  bal_b : Subsystem
  bal_g : Subsystem
  bal_r : Subsystem
  hsdelay : xbsIndex_r4/Delay  en=on  latency=3  dbl_ovrd=off  reg_retiming=on  block_type=delay
      settings: infoedit="Delay line having  configurable length.<P><P>Hardware notes: A delay line is a chain, each link of which is an SRL16 followed by a flip-flop. If register retiming is enabled, the delay line is a chain of flip-flops."  xl_area=[0, 0, 0, 0, 0, 0, 0]  block_version=VER_STRING_GOES_HERE
  vsdelay : xbsIndex_r4/Delay  en=on  latency=3  dbl_ovrd=off  reg_retiming=on  block_type=delay
      settings: infoedit="Delay line having  configurable length.<P><P>Hardware notes: A delay line is a chain, each link of which is an SRL16 followed by a flip-flop. If register retiming is enabled, the delay line is a chain of flip-flops."  xl_area=[0, 0, 0, 0, 0, 0, 0]  block_version=VER_STRING_GOES_HERE
  vso : Outport
  hso : Outport  Port=2
  ro : Outport  Port=3
  go : Outport  Port=4
  bo : Outport  Port=5
  eo : Outport  Port=6
  wires:
  hs/1 -> hsdelay/1
  Inverter1/1 -> bal_b/2(bypass), bal_g/2(bypass), bal_r/2(bypass)
  Constant/1 -> Inverter1/1
  Convert1/1 -> bal_b/3(update), bal_g/3(update), bal_r/3(update)
  Inverter2/1 -> Convert1/1
  vs/1 -> Inverter2/1, vsdelay/1
  bal_b/1(v_out) -> bo/1
  b/1 -> bal_b/1(v_in)
  bal_g/1(v_out) -> go/1
  g/1 -> bal_g/1(v_in)
  bal_r/1(v_out) -> ro/1
  r/1 -> bal_r/1(v_in)
  e/1 -> vsdelay/2, hsdelay/2, eo/1
  vsdelay/1 -> vso/1
  hsdelay/1 -> hso/1
